simulink model "gm_FOC"  (R2020a)
settings: Solver=FixedStepAuto  StartTime=0.0  StopTime=10.0  RelTol=1e-3
libraries: hdlmdlgenlib x12
(part 1 of 2)
settings Model: Creator=black  LastModifiedBy=black
settings OptimizationCC: BlockReduction=off  ConditionallyExecuteInputs=off
settings DebuggingCC: InheritedTsInSrcMsg=none  SingleTaskRateTransMsg=error

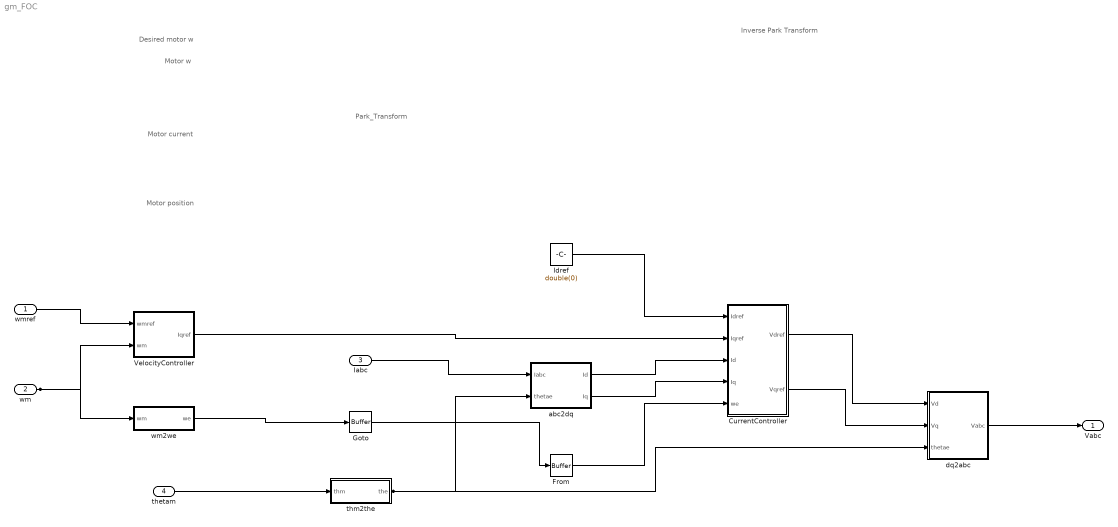
== system gm_FOC ==
  note: Motor position
  note: Motor current
  note: Desired motor w
  note: Motor w
  note: Park_Transform
  note: Inverse Park Transform
  wmref : Inport  OutDataTypeStr=double  Unit=rad/sec  PortDimensions=1  SampleTime=10000
  wm : Inport  Port=2  OutDataTypeStr=double  Unit=rad/sec  PortDimensions=1  SampleTime=10000
  Iabc : Inport  Port=3  OutDataTypeStr=single  Unit=A  PortDimensions=[3]  SampleTime=10000
  thetam : Inport  Port=4  OutDataTypeStr=double  Unit=rad  PortDimensions=1  SampleTime=10000
  CurrentController : Subsystem
  From : hdlmdlgenlib/Buffer
      settings: SourceProductBaseCode=SL
  Goto : hdlmdlgenlib/Buffer
      settings: SourceProductBaseCode=SL
  Idref : Constant  Value=double(0)  OutDataTypeStr=double  SampleTime=10000
  VelocityController : Subsystem
  abc2dq : Subsystem
  dq2abc : Subsystem
  thm2the : Subsystem
  wm2we : Subsystem
  Vabc : Outport  Unit=V  PortDimensions=3  VectorParamsAs1DForOutWhenUnconnected=off
  wires:
  wmref/1 -> VelocityController/1(wmref)
  wm/1 -> VelocityController/2(wm), wm2we/1(wm)
  Iabc/1 -> abc2dq/1(Iabc)
  thetam/1 -> thm2the/1(thm)
  CurrentController/1(Vdref) -> dq2abc/1(Vd)
  CurrentController/2(Vqref) -> dq2abc/2(Vq)
  From/1 -> CurrentController/5(we)
  Idref/1 -> CurrentController/1(Idref)
  VelocityController/1(Iqref) -> CurrentController/2(Iqref)
  abc2dq/1(Id) -> CurrentController/3(Id)
  abc2dq/2(Iq) -> CurrentController/4(Iq)
  dq2abc/1(Vabc) -> Vabc/1
  thm2the/1(the) -> abc2dq/2(thetae), dq2abc/3(thetae)
  wm2we/1(we) -> Goto/1
  Goto/1 -> From/1

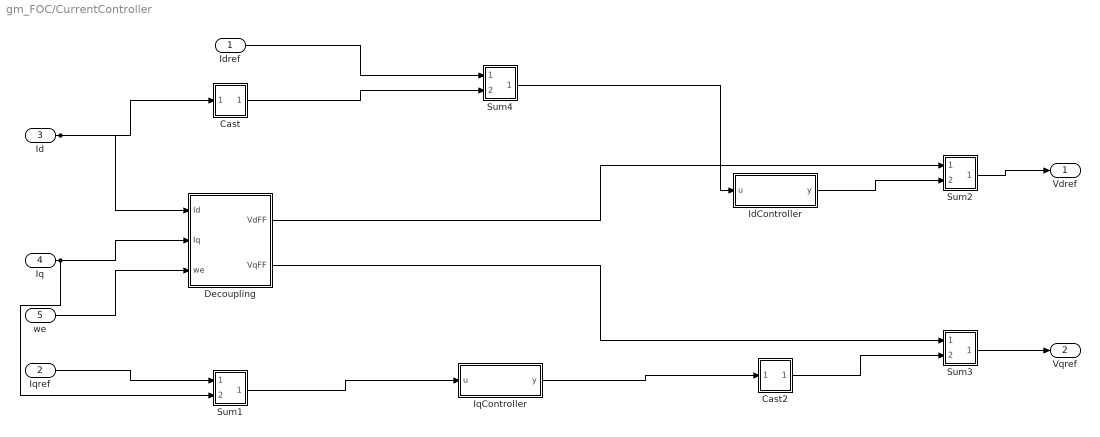
== system gm_FOC/CurrentController ==
  Idref : Inport  OutDataTypeStr=double  PortDimensions=1  SampleTime=10000
  Iqref : Inport  Port=2  OutDataTypeStr=single  PortDimensions=1  SampleTime=10000
  Id : Inport  Port=3  OutDataTypeStr=single  PortDimensions=1  SampleTime=10000
  Iq : Inport  Port=4  OutDataTypeStr=single  PortDimensions=1  SampleTime=10000
  we : Inport  Port=5  OutDataTypeStr=double  PortDimensions=1  SampleTime=10000
  Cast : Subsystem
      mask Display: disp('NFP\nconv');
  Cast2 : Subsystem
      mask Display: disp('NFP\nconv');
  Decoupling : Subsystem
  IdController : Subsystem
  IqController : Subsystem
  Sum1 : Subsystem
      mask Display: disp('NFP\nadd');
  Sum2 : Subsystem
      mask Display: disp('NFP\nadd');
  Sum3 : Subsystem
      mask Display: disp('NFP\nadd');
  Sum4 : Subsystem
      mask Display: disp('NFP\nadd');
  Vdref : Outport  VectorParamsAs1DForOutWhenUnconnected=off
  Vqref : Outport  Port=2  VectorParamsAs1DForOutWhenUnconnected=off
  wires:
  Idref/1 -> Sum4/1(In1)
  Iqref/1 -> Sum1/1(In1)
  Id/1 -> Cast/1(In1), Decoupling/1(Id)
  Iq/1 -> Sum1/2(In2), Decoupling/2(Iq)
  we/1 -> Decoupling/3(we)
  Decoupling/1(VdFF) -> Sum2/1(In1)
  Decoupling/2(VqFF) -> Sum3/1(In1)
  IdController/1(y) -> Sum2/2(In2)
  IqController/1(y) -> Cast2/1(In1)
  Cast/1(Out1) -> Sum4/2(In2)
  Cast2/1(Out1) -> Sum3/2(In2)
  Sum1/1(Out1) -> IqController/1(u)
  Sum2/1(Out1) -> Vdref/1
  Sum3/1(Out1) -> Vqref/1
  Sum4/1(Out1) -> IdController/1(u)

== system gm_FOC/VelocityController ==
  wmref : Inport  OutDataTypeStr=double  PortDimensions=1  SampleTime=10000
  wm : Inport  Port=2  OutDataTypeStr=double  PortDimensions=1  SampleTime=10000
  Cast : Subsystem
      mask Display: disp('NFP\nconv');
  Gain : Subsystem
      mask Display: disp('NFP\nmul');
  Gain_const : Constant  Value=single(3.3333332538604736)  OutDataTypeStr=single  SampleTime=10000
  PIDController : Subsystem
  Sum : Subsystem
      mask Display: disp('NFP\nadd');
  Iqref : Outport  VectorParamsAs1DForOutWhenUnconnected=off
  wires:
  wmref/1 -> Sum/1(In1)
  wm/1 -> Sum/2(In2)
  PIDController/1(y) -> Cast/1(In1)
  Gain_const/1 -> Gain/1(In1)
  Cast/1(Out1) -> Gain/2(In2)
  Sum/1(Out1) -> PIDController/1(u)
  Gain/1(Out1) -> Iqref/1

== system gm_FOC/abc2dq ==
  Iabc : Inport  OutDataTypeStr=single  PortDimensions=[3]  SampleTime=10000
  thetae : Inport  Port=2  OutDataTypeStr=single  PortDimensions=1  SampleTime=10000
  Park Transform : Subsystem  mask(Park Transform){AxisAlignment=D-axis, PowerInvariant=off}
      mask prompts: AxisAlignment "physmod:ee:library:comments:control:eeTransforms:PhaseaAxisAlignment_MP"; PowerInvariant "physmod:ee:library:comments:control:eeTransforms:PowerInvariant_MP"
      mask help: physmod:ee:library:comments:control:eeTransforms:ParkTransform_MD
      mask Help: web(nesl_help(gcbh))
      mask TypeOptions AxisAlignment: physmod:ee:library:comments:control:eeTransforms:Q0x2DAxis_PV | physmod:ee:library:comments:control:eeTransforms:D0x2DAxis_PV
      mask Display: ee.mask.drawParkTransform();
  Terminator : Terminator
  t : Demux  Outputs=3
  Id : Outport  VectorParamsAs1DForOutWhenUnconnected=off
  Iq : Outport  Port=2  VectorParamsAs1DForOutWhenUnconnected=off
  wires:
  Iabc/1 -> Park Transform/1(abc)
  thetae/1 -> Park Transform/2(theta)
  Park Transform/1(dq0) -> t/1
  t/1 -> Id/1
  t/2 -> Iq/1
  t/3 -> Terminator/1

== system gm_FOC/dq2abc ==
  Vd : Inport  OutDataTypeStr=double  PortDimensions=1  SampleTime=10000
  Vq : Inport  Port=2  OutDataTypeStr=double  PortDimensions=1  SampleTime=10000
  thetae : Inport  Port=3  OutDataTypeStr=single  PortDimensions=1  SampleTime=10000
  Cast : Subsystem
      mask Display: disp('NFP\nconv');
  Constant : Constant  Value=double(0)  OutDataTypeStr=double  SampleTime=10000
  Inverse Park Transform : Subsystem  mask(Inverse Park Transform){AxisAlignment=D-axis, PowerInvariant=off}
      mask prompts: AxisAlignment "physmod:ee:library:comments:control:eeTransforms:PhaseaAxisAlignment_MP"; PowerInvariant "physmod:ee:library:comments:control:eeTransforms:PowerInvariant_MP"
      mask help: physmod:ee:library:comments:control:eeTransforms:InverseParkTransform_MD
      mask Help: web(nesl_help(gcbh))
      mask TypeOptions AxisAlignment: physmod:ee:library:comments:control:eeTransforms:Q0x2DAxis_PV | physmod:ee:library:comments:control:eeTransforms:D0x2DAxis_PV
      mask Display: ee.mask.drawInverseParkTransform();
  mux : Mux  Inputs=3
  Vabc : Outport  Unit=V  PortDimensions=3  VectorParamsAs1DForOutWhenUnconnected=off
  wires:
  Vd/1 -> mux/1
  Vq/1 -> mux/2
  thetae/1 -> Inverse Park Transform/2(theta)
  Constant/1 -> mux/3
  Inverse Park Transform/1(abc) -> Vabc/1
  mux/1 -> Cast/1(In1)
  Cast/1(Out1) -> Inverse Park Transform/1(dq0)

== system gm_FOC/thm2the ==
  thm : Inport  OutDataTypeStr=double  PortDimensions=1  SampleTime=10000
  Cast : Subsystem
      mask Display: disp('NFP\nconv');
  Cast1 : Subsystem
      mask Display: disp('NFP\nconv');
  Constant : Constant  Value=double(6.283185307179586)  OutDataTypeStr=double  SampleTime=10000
  Mod : Subsystem
      mask Display: disp('NFP\nmath2');
  PolePairs : Subsystem
      mask Display: disp('NFP\ngain_pow2');
  the : Outport  VectorParamsAs1DForOutWhenUnconnected=off
  wires:
  thm/1 -> PolePairs/1(In1)
  Constant/1 -> Cast/1(In1)
  PolePairs/1(Out1) -> Cast1/1(In1)
  Cast/1(Out1) -> Mod/2(In2)
  Cast1/1(Out1) -> Mod/1(In1)
  Mod/1(Out1) -> the/1

== system gm_FOC/wm2we ==
  wm : Inport  OutDataTypeStr=double  PortDimensions=1  SampleTime=10000
  PolePairs : Subsystem
      mask Display: disp('NFP\ngain_pow2');
  we : Outport  VectorParamsAs1DForOutWhenUnconnected=off
  wires:
  wm/1 -> PolePairs/1(In1)
  PolePairs/1(Out1) -> we/1

== system gm_FOC/CurrentController/Cast ==
  In1 : Inport
  Cast : DataTypeConversion  OutDataTypeStr=double  RndMeth=Nearest  SampleTime=10000
  Out1 : Outport
  wires:
  In1/1 -> Cast/1
  Cast/1 -> Out1/1

== system gm_FOC/CurrentController/Cast2 ==
  In1 : Inport
  Cast2 : DataTypeConversion  OutDataTypeStr=double  RndMeth=Nearest  SampleTime=10000
  Out1 : Outport
  wires:
  In1/1 -> Cast2/1
  Cast2/1 -> Out1/1

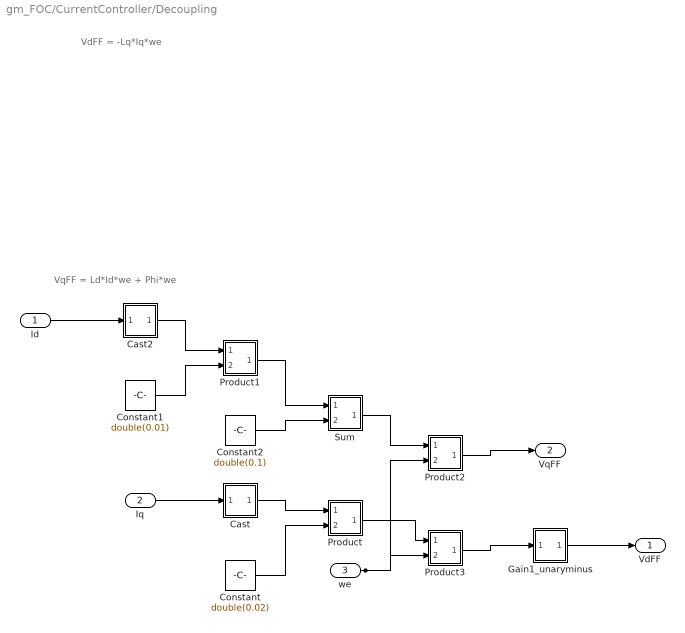
== system gm_FOC/CurrentController/Decoupling ==
  note: VdFF = -Lq*Iq*we
  note: VqFF = Ld*Id*we + Phi*we
  Id : Inport  OutDataTypeStr=single  PortDimensions=1  SampleTime=10000
  Iq : Inport  Port=2  OutDataTypeStr=single  PortDimensions=1  SampleTime=10000
  we : Inport  Port=3  OutDataTypeStr=double  PortDimensions=1  SampleTime=10000
  Cast : Subsystem
      mask Display: disp('NFP\nconv');
  Cast2 : Subsystem
      mask Display: disp('NFP\nconv');
  Constant : Constant  Value=double(0.02)  OutDataTypeStr=double  SampleTime=10000
  Constant1 : Constant  Value=double(0.01)  OutDataTypeStr=double  SampleTime=10000
  Constant2 : Constant  Value=double(0.1)  OutDataTypeStr=double  SampleTime=10000
  Gain1_unaryminus : Subsystem
      mask Display: disp('NFP\numinus');
  Product : Subsystem
      mask Display: disp('NFP\nmul');
  Product1 : Subsystem
      mask Display: disp('NFP\nmul');
  Product2 : Subsystem
      mask Display: disp('NFP\nmul');
  Product3 : Subsystem
      mask Display: disp('NFP\nmul');
  Sum : Subsystem
      mask Display: disp('NFP\nadd');
  VdFF : Outport  VectorParamsAs1DForOutWhenUnconnected=off
  VqFF : Outport  Port=2  VectorParamsAs1DForOutWhenUnconnected=off
  wires:
  Id/1 -> Cast2/1(In1)
  Iq/1 -> Cast/1(In1)
  we/1 -> Product3/2(In2), Product2/2(In2)
  Constant/1 -> Product/2(In2)
  Constant1/1 -> Product1/2(In2)
  Constant2/1 -> Sum/2(In2)
  Gain1_unaryminus/1(Out1) -> VdFF/1
  Cast/1(Out1) -> Product/1(In1)
  Cast2/1(Out1) -> Product1/1(In1)
  Product/1(Out1) -> Product3/1(In1)
  Product1/1(Out1) -> Sum/1(In1)
  Product2/1(Out1) -> VqFF/1
  Product3/1(Out1) -> Gain1_unaryminus/1(In1)
  Sum/1(Out1) -> Product2/1(In1)

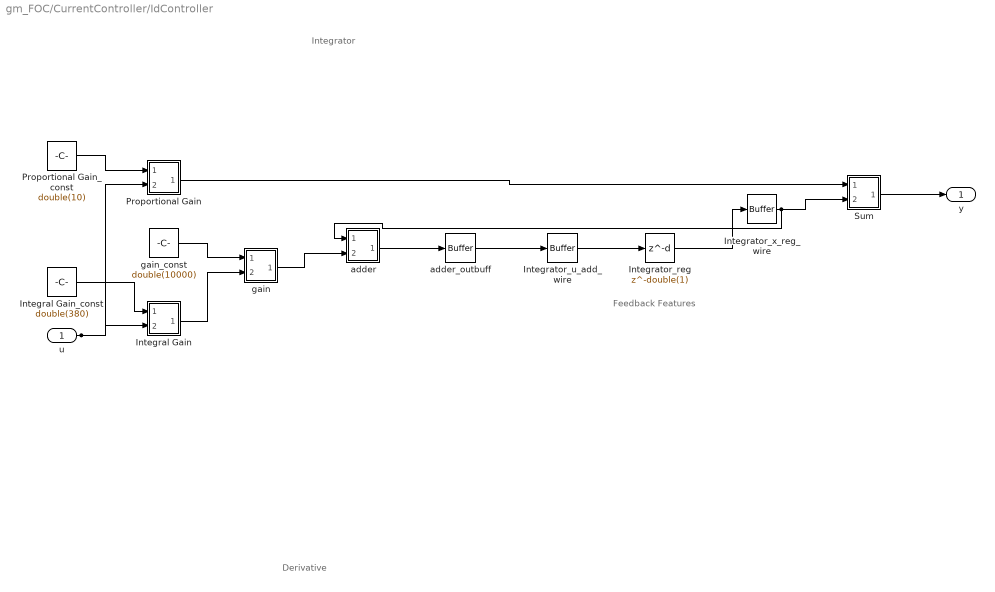
== system gm_FOC/CurrentController/IdController ==
  note: Feedback Features
  note: Derivative
  note: Integrator
  u : Inport  OutDataTypeStr=double  SampleTime=10000
  Integral Gain : Subsystem
      mask Display: disp('NFP\nmul');
  Integral Gain_const : Constant  Value=double(380)  OutDataTypeStr=double  SampleTime=10000
  Integrator_reg : Delay  DelayLength=double(1)  InitialCondition=0  SampleTime=10000
  Integrator_u_add_wire : hdlmdlgenlib/Buffer
      settings: SourceProductBaseCode=SL
  Integrator_x_reg_wire : hdlmdlgenlib/Buffer
      settings: SourceProductBaseCode=SL
  Proportional Gain : Subsystem
      mask Display: disp('NFP\nmul');
  Proportional Gain_const : Constant  Value=double(10)  OutDataTypeStr=double  SampleTime=10000
  Sum : Subsystem
      mask Display: disp('NFP\nadd');
  adder : Subsystem
      mask Display: disp('NFP\nadd');
  adder_outbuff : hdlmdlgenlib/Buffer
      settings: SourceProductBaseCode=SL
  gain : Subsystem
      mask Display: disp('NFP\nmul');
  gain_const : Constant  Value=double(10000)  OutDataTypeStr=double  SampleTime=10000
  y : Outport
  wires:
  u/1 -> Proportional Gain/2(In2), Integral Gain/2(In2)
  Integrator_x_reg_wire/1 -> Sum/2(In2), adder/1(In1)
  adder_outbuff/1 -> Integrator_u_add_wire/1
  Integrator_u_add_wire/1 -> Integrator_reg/1
  Integrator_reg/1 -> Integrator_x_reg_wire/1
  Integral Gain_const/1 -> Integral Gain/1(In1)
  gain_const/1 -> gain/1(In1)
  Proportional Gain_const/1 -> Proportional Gain/1(In1)
  adder/1(Out1) -> adder_outbuff/1
  Sum/1(Out1) -> y/1
  Integral Gain/1(Out1) -> gain/2(In2)
  gain/1(Out1) -> adder/2(In2)
  Proportional Gain/1(Out1) -> Sum/1(In1)

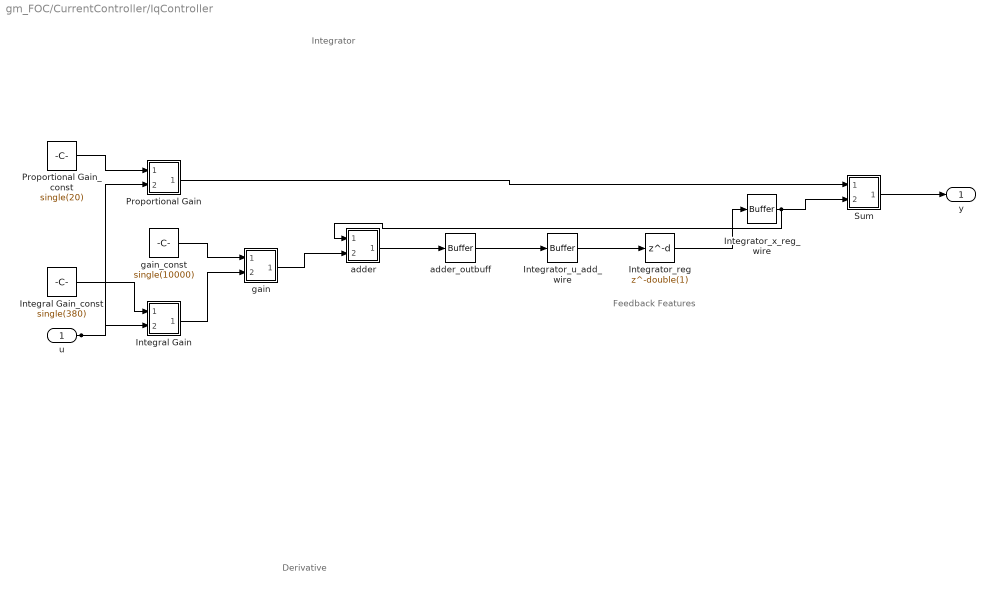
== system gm_FOC/CurrentController/IqController ==
  note: Feedback Features
  note: Derivative
  note: Integrator
  u : Inport  OutDataTypeStr=single  SampleTime=10000
  Integral Gain : Subsystem
      mask Display: disp('NFP\nmul');
  Integral Gain_const : Constant  Value=single(380)  OutDataTypeStr=single  SampleTime=10000
  Integrator_reg : Delay  DelayLength=double(1)  InitialCondition=0  SampleTime=10000
  Integrator_u_add_wire : hdlmdlgenlib/Buffer
      settings: SourceProductBaseCode=SL
  Integrator_x_reg_wire : hdlmdlgenlib/Buffer
      settings: SourceProductBaseCode=SL
  Proportional Gain : Subsystem
      mask Display: disp('NFP\nmul');
  Proportional Gain_const : Constant  Value=single(20)  OutDataTypeStr=single  SampleTime=10000
  Sum : Subsystem
      mask Display: disp('NFP\nadd');
  adder : Subsystem
      mask Display: disp('NFP\nadd');
  adder_outbuff : hdlmdlgenlib/Buffer
      settings: SourceProductBaseCode=SL
  gain : Subsystem
      mask Display: disp('NFP\nmul');
  gain_const : Constant  Value=single(10000)  OutDataTypeStr=single  SampleTime=10000
  y : Outport
  wires:
  u/1 -> Proportional Gain/2(In2), Integral Gain/2(In2)
  Integrator_x_reg_wire/1 -> Sum/2(In2), adder/1(In1)
  adder_outbuff/1 -> Integrator_u_add_wire/1
  Integrator_u_add_wire/1 -> Integrator_reg/1
  Integrator_reg/1 -> Integrator_x_reg_wire/1
  Integral Gain_const/1 -> Integral Gain/1(In1)
  gain_const/1 -> gain/1(In1)
  Proportional Gain_const/1 -> Proportional Gain/1(In1)
  adder/1(Out1) -> adder_outbuff/1
  Sum/1(Out1) -> y/1
  Integral Gain/1(Out1) -> gain/2(In2)
  gain/1(Out1) -> adder/2(In2)
  Proportional Gain/1(Out1) -> Sum/1(In1)

== system gm_FOC/CurrentController/Sum1 ==
  In1 : Inport
  In2 : Inport  Port=2
  Sum1 : Sum  Inputs=+-  OutDataTypeStr=single  SampleTime=10000
  Out1 : Outport
  wires:
  In1/1 -> Sum1/1
  In2/1 -> Sum1/2
  Sum1/1 -> Out1/1

== system gm_FOC/CurrentController/Sum2 ==
  In1 : Inport
  In2 : Inport  Port=2
  Sum2 : Sum  OutDataTypeStr=double  SampleTime=10000
  Out1 : Outport
  wires:
  In1/1 -> Sum2/1
  In2/1 -> Sum2/2
  Sum2/1 -> Out1/1

== system gm_FOC/CurrentController/Sum3 ==
  In1 : Inport
  In2 : Inport  Port=2
  Sum3 : Sum  OutDataTypeStr=double  SampleTime=10000
  Out1 : Outport
  wires:
  In1/1 -> Sum3/1
  In2/1 -> Sum3/2
  Sum3/1 -> Out1/1

== system gm_FOC/CurrentController/Sum4 ==
  In1 : Inport
  In2 : Inport  Port=2
  Sum4 : Sum  Inputs=+-  OutDataTypeStr=double  SampleTime=10000
  Out1 : Outport
  wires:
  In1/1 -> Sum4/1
  In2/1 -> Sum4/2
  Sum4/1 -> Out1/1

== system gm_FOC/VelocityController/Cast ==
  In1 : Inport
  Cast : DataTypeConversion  OutDataTypeStr=single  RndMeth=Nearest  SampleTime=10000
  Out1 : Outport
  wires:
  In1/1 -> Cast/1
  Cast/1 -> Out1/1

== system gm_FOC/VelocityController/Gain ==
  In1 : Inport
  In2 : Inport  Port=2
  Gain : Product  Inputs=**  OutDataTypeStr=single  SampleTime=10000
  Out1 : Outport
  wires:
  In1/1 -> Gain/1
  In2/1 -> Gain/2
  Gain/1 -> Out1/1

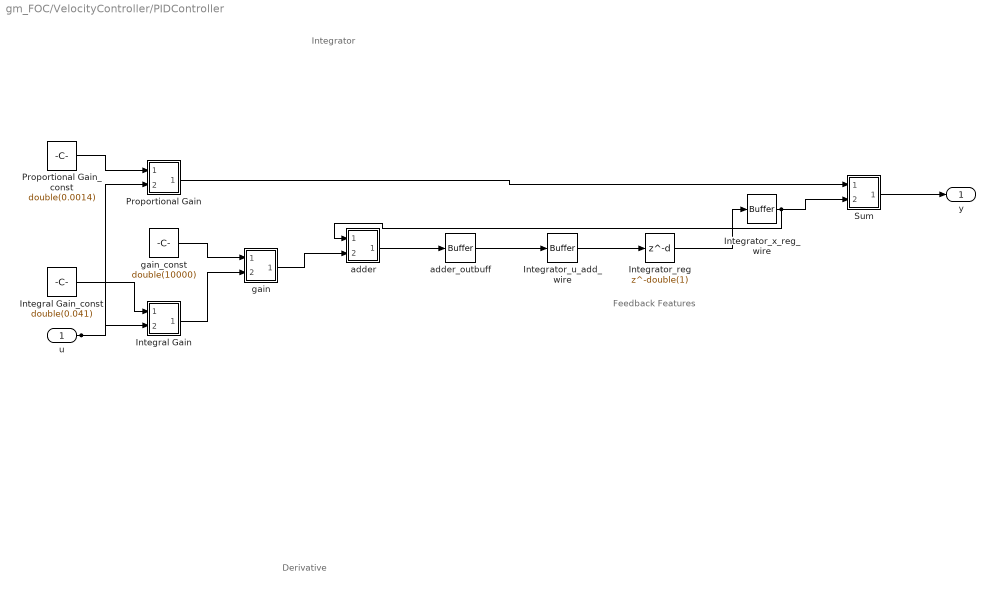
== system gm_FOC/VelocityController/PIDController ==
  note: Feedback Features
  note: Derivative
  note: Integrator
  u : Inport  OutDataTypeStr=double  SampleTime=10000
  Integral Gain : Subsystem
      mask Display: disp('NFP\nmul');
  Integral Gain_const : Constant  Value=double(0.041)  OutDataTypeStr=double  SampleTime=10000
  Integrator_reg : Delay  DelayLength=double(1)  InitialCondition=0  SampleTime=10000
  Integrator_u_add_wire : hdlmdlgenlib/Buffer
      settings: SourceProductBaseCode=SL
  Integrator_x_reg_wire : hdlmdlgenlib/Buffer
      settings: SourceProductBaseCode=SL
  Proportional Gain : Subsystem
      mask Display: disp('NFP\nmul');
  Proportional Gain_const : Constant  Value=double(0.0014)  OutDataTypeStr=double  SampleTime=10000
  Sum : Subsystem
      mask Display: disp('NFP\nadd');
  adder : Subsystem
      mask Display: disp('NFP\nadd');
  adder_outbuff : hdlmdlgenlib/Buffer
      settings: SourceProductBaseCode=SL
  gain : Subsystem
      mask Display: disp('NFP\nmul');
  gain_const : Constant  Value=double(10000)  OutDataTypeStr=double  SampleTime=10000
  y : Outport
  wires:
  u/1 -> Proportional Gain/2(In2), Integral Gain/2(In2)
  Integrator_x_reg_wire/1 -> Sum/2(In2), adder/1(In1)
  adder_outbuff/1 -> Integrator_u_add_wire/1
  Integrator_u_add_wire/1 -> Integrator_reg/1
  Integrator_reg/1 -> Integrator_x_reg_wire/1
  Integral Gain_const/1 -> Integral Gain/1(In1)
  gain_const/1 -> gain/1(In1)
  Proportional Gain_const/1 -> Proportional Gain/1(In1)
  adder/1(Out1) -> adder_outbuff/1
  Sum/1(Out1) -> y/1
  Integral Gain/1(Out1) -> gain/2(In2)
  gain/1(Out1) -> adder/2(In2)
  Proportional Gain/1(Out1) -> Sum/1(In1)

== system gm_FOC/VelocityController/Sum ==
  In1 : Inport
  In2 : Inport  Port=2
  Sum : Sum  Inputs=+-  OutDataTypeStr=double  SampleTime=10000
  Out1 : Outport
  wires:
  In1/1 -> Sum/1
  In2/1 -> Sum/2
  Sum/1 -> Out1/1

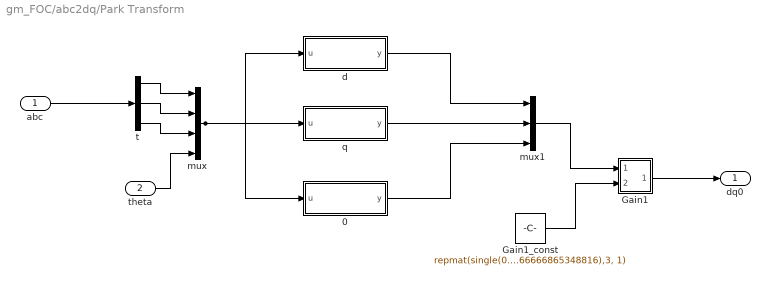
== system gm_FOC/abc2dq/Park Transform ==
  abc : Inport  OutDataTypeStr=single  PortDimensions=[3]  SampleTime=10000
  theta : Inport  Port=2  OutDataTypeStr=single  SampleTime=10000
  0 : Subsystem
  Gain1 : Subsystem
      mask Display: disp('NFP\nmul');
  Gain1_const : Constant  Value=repmat(single(0.6666666865348816),3, 1)  OutDataTypeStr=single  SampleTime=10000
  d : Subsystem
  mux : Mux
  mux1 : Mux  Inputs=3
  q : Subsystem
  t : Demux  Outputs=3
  dq0 : Outport
  wires:
  abc/1 -> t/1
  theta/1 -> mux/4
  0/1(y) -> mux1/3
  mux/1 -> q/1(u), d/1(u), 0/1(u)
  mux1/1 -> Gain1/1(In1)
  d/1(y) -> mux1/1
  q/1(y) -> mux1/2
  t/1 -> mux/1
  t/2 -> mux/2
  t/3 -> mux/3
  Gain1_const/1 -> Gain1/2(In2)
  Gain1/1(Out1) -> dq0/1

== system gm_FOC/dq2abc/Cast ==
  In1 : Inport
  Cast : DataTypeConversion  OutDataTypeStr=single  RndMeth=Nearest  SampleTime=10000
  Out1 : Outport
  wires:
  In1/1 -> Cast/1
  Cast/1 -> Out1/1

== system gm_FOC/dq2abc/Inverse Park Transform ==
  dq0 : Inport  OutDataTypeStr=single  PortDimensions=[3]  SampleTime=10000
  theta : Inport  Port=2  OutDataTypeStr=single  SampleTime=10000
  Gain1_unary : hdlmdlgenlib/Buffer
      settings: SourceProductBaseCode=SL
  a : Subsystem
  b : Subsystem
  c : Subsystem
  mux : Mux
  mux1 : Mux  Inputs=3
  t : Demux  Outputs=3
  abc : Outport
  wires:
  dq0/1 -> t/1
  theta/1 -> mux/4
  Gain1_unary/1 -> abc/1
  mux/1 -> c/1(u), b/1(u), a/1(u)
  mux1/1 -> Gain1_unary/1
  a/1(y) -> mux1/1
  b/1(y) -> mux1/2
  c/1(y) -> mux1/3
  t/1 -> mux/1
  t/2 -> mux/2
  t/3 -> mux/3

== system gm_FOC/thm2the/Cast ==
  In1 : Inport
  Cast : DataTypeConversion  OutDataTypeStr=single  RndMeth=Nearest  SampleTime=10000
  Out1 : Outport
  wires:
  In1/1 -> Cast/1
  Cast/1 -> Out1/1

== system gm_FOC/thm2the/Cast1 ==
  In1 : Inport
  Cast1 : DataTypeConversion  OutDataTypeStr=single  RndMeth=Nearest  SampleTime=10000
  Out1 : Outport
  wires:
  In1/1 -> Cast1/1
  Cast1/1 -> Out1/1

== system gm_FOC/thm2the/Mod ==
  In1 : Inport
  In2 : Inport  Port=2
  Mod : Math  Operator=mod  SampleTime=10000  SaturateOnIntegerOverflow=on
  Out1 : Outport
  wires:
  In1/1 -> Mod/1
  In2/1 -> Mod/2
  Mod/1 -> Out1/1

== system gm_FOC/thm2the/PolePairs ==
  In1 : Inport
  PolePairs : Gain  Gain=double(2)
  Out1 : Outport
  wires:
  In1/1 -> PolePairs/1
  PolePairs/1 -> Out1/1

== system gm_FOC/wm2we/PolePairs ==
  In1 : Inport
  PolePairs : Gain  Gain=double(2)
  Out1 : Outport
  wires:
  In1/1 -> PolePairs/1
  PolePairs/1 -> Out1/1

== system gm_FOC/CurrentController/Decoupling/Cast ==
  In1 : Inport
  Cast : DataTypeConversion  OutDataTypeStr=double  RndMeth=Nearest  SampleTime=10000
  Out1 : Outport
  wires:
  In1/1 -> Cast/1
  Cast/1 -> Out1/1

== system gm_FOC/CurrentController/Decoupling/Cast2 ==
  In1 : Inport
  Cast2 : DataTypeConversion  OutDataTypeStr=double  RndMeth=Nearest  SampleTime=10000
  Out1 : Outport
  wires:
  In1/1 -> Cast2/1
  Cast2/1 -> Out1/1

== system gm_FOC/CurrentController/Decoupling/Gain1_unaryminus ==
  In1 : Inport
  Gain1_unaryminus : UnaryMinus  SampleTime=10000
  Out1 : Outport
  wires:
  In1/1 -> Gain1_unaryminus/1
  Gain1_unaryminus/1 -> Out1/1

== system gm_FOC/CurrentController/Decoupling/Product ==
  In1 : Inport
  In2 : Inport  Port=2
  Product : Product  Inputs=**  OutDataTypeStr=double  SampleTime=10000
  Out1 : Outport
  wires:
  In1/1 -> Product/1
  In2/1 -> Product/2
  Product/1 -> Out1/1

== system gm_FOC/CurrentController/Decoupling/Product1 ==
  In1 : Inport
  In2 : Inport  Port=2
  Product1 : Product  Inputs=**  OutDataTypeStr=double  SampleTime=10000
  Out1 : Outport
  wires:
  In1/1 -> Product1/1
  In2/1 -> Product1/2
  Product1/1 -> Out1/1

== system gm_FOC/CurrentController/Decoupling/Product2 ==
  In1 : Inport
  In2 : Inport  Port=2
  Product2 : Product  Inputs=**  OutDataTypeStr=double  SampleTime=10000
  Out1 : Outport
  wires:
  In1/1 -> Product2/1
  In2/1 -> Product2/2
  Product2/1 -> Out1/1

== system gm_FOC/CurrentController/Decoupling/Product3 ==
  In1 : Inport
  In2 : Inport  Port=2
  Product3 : Product  Inputs=**  OutDataTypeStr=double  SampleTime=10000
  Out1 : Outport
  wires:
  In1/1 -> Product3/1
  In2/1 -> Product3/2
  Product3/1 -> Out1/1

== system gm_FOC/CurrentController/Decoupling/Sum ==
  In1 : Inport
  In2 : Inport  Port=2
  Sum : Sum  OutDataTypeStr=double  SampleTime=10000
  Out1 : Outport
  wires:
  In1/1 -> Sum/1
  In2/1 -> Sum/2
  Sum/1 -> Out1/1

== system gm_FOC/CurrentController/IdController/Integral Gain ==
  In1 : Inport
  In2 : Inport  Port=2
  Integral Gain : Product  Inputs=**  OutDataTypeStr=double  SampleTime=10000
  Out1 : Outport
  wires:
  In1/1 -> Integral Gain/1
  In2/1 -> Integral Gain/2
  Integral Gain/1 -> Out1/1

== system gm_FOC/CurrentController/IdController/Proportional Gain ==
  In1 : Inport
  In2 : Inport  Port=2
  Proportional Gain : Product  Inputs=**  OutDataTypeStr=double  SampleTime=10000
  Out1 : Outport
  wires:
  In1/1 -> Proportional Gain/1
  In2/1 -> Proportional Gain/2
  Proportional Gain/1 -> Out1/1

== system gm_FOC/CurrentController/IdController/Sum ==
  In1 : Inport
  In2 : Inport  Port=2
  Sum : Sum  OutDataTypeStr=double  SampleTime=10000
  Out1 : Outport
  wires:
  In1/1 -> Sum/1
  In2/1 -> Sum/2
  Sum/1 -> Out1/1

== system gm_FOC/CurrentController/IdController/adder ==
  In1 : Inport
  In2 : Inport  Port=2
  adder : Sum  OutDataTypeStr=double  SampleTime=10000
  Out1 : Outport
  wires:
  In1/1 -> adder/1
  In2/1 -> adder/2
  adder/1 -> Out1/1

== system gm_FOC/CurrentController/IdController/gain ==
  In1 : Inport
  In2 : Inport  Port=2
  gain : Product  Inputs=**  OutDataTypeStr=double  SampleTime=10000
  Out1 : Outport
  wires:
  In1/1 -> gain/1
  In2/1 -> gain/2
  gain/1 -> Out1/1

== system gm_FOC/CurrentController/IqController/Integral Gain ==
  In1 : Inport
  In2 : Inport  Port=2
  Integral Gain : Product  Inputs=**  OutDataTypeStr=single  SampleTime=10000
  Out1 : Outport
  wires:
  In1/1 -> Integral Gain/1
  In2/1 -> Integral Gain/2
  Integral Gain/1 -> Out1/1

== system gm_FOC/CurrentController/IqController/Proportional Gain ==
  In1 : Inport
  In2 : Inport  Port=2
  Proportional Gain : Product  Inputs=**  OutDataTypeStr=single  SampleTime=10000
  Out1 : Outport
  wires:
  In1/1 -> Proportional Gain/1
  In2/1 -> Proportional Gain/2
  Proportional Gain/1 -> Out1/1

== system gm_FOC/CurrentController/IqController/Sum ==
  In1 : Inport
  In2 : Inport  Port=2
  Sum : Sum  OutDataTypeStr=single  SampleTime=10000
  Out1 : Outport
  wires:
  In1/1 -> Sum/1
  In2/1 -> Sum/2
  Sum/1 -> Out1/1

== system gm_FOC/CurrentController/IqController/adder ==
  In1 : Inport
  In2 : Inport  Port=2
  adder : Sum  OutDataTypeStr=single  SampleTime=10000
  Out1 : Outport
  wires:
  In1/1 -> adder/1
  In2/1 -> adder/2
  adder/1 -> Out1/1

== system gm_FOC/CurrentController/IqController/gain ==
  In1 : Inport
  In2 : Inport  Port=2
  gain : Product  Inputs=**  OutDataTypeStr=single  SampleTime=10000
  Out1 : Outport
  wires:
  In1/1 -> gain/1
  In2/1 -> gain/2
  gain/1 -> Out1/1

== system gm_FOC/VelocityController/PIDController/Integral Gain ==
  In1 : Inport
  In2 : Inport  Port=2
  Integral Gain : Product  Inputs=**  OutDataTypeStr=double  SampleTime=10000
  Out1 : Outport
  wires:
  In1/1 -> Integral Gain/1
  In2/1 -> Integral Gain/2
  Integral Gain/1 -> Out1/1

== system gm_FOC/VelocityController/PIDController/Proportional Gain ==
  In1 : Inport
  In2 : Inport  Port=2
  Proportional Gain : Product  Inputs=**  OutDataTypeStr=double  SampleTime=10000
  Out1 : Outport
  wires:
  In1/1 -> Proportional Gain/1
  In2/1 -> Proportional Gain/2
  Proportional Gain/1 -> Out1/1

== system gm_FOC/VelocityController/PIDController/Sum ==
  In1 : Inport
  In2 : Inport  Port=2
  Sum : Sum  OutDataTypeStr=double  SampleTime=10000
  Out1 : Outport
  wires:
  In1/1 -> Sum/1
  In2/1 -> Sum/2
  Sum/1 -> Out1/1

== system gm_FOC/VelocityController/PIDController/adder ==
  In1 : Inport
  In2 : Inport  Port=2
  adder : Sum  OutDataTypeStr=double  SampleTime=10000
  Out1 : Outport
  wires:
  In1/1 -> adder/1
  In2/1 -> adder/2
  adder/1 -> Out1/1

== system gm_FOC/VelocityController/PIDController/gain ==
  In1 : Inport
  In2 : Inport  Port=2
  gain : Product  Inputs=**  OutDataTypeStr=double  SampleTime=10000
  Out1 : Outport
  wires:
  In1/1 -> gain/1
  In2/1 -> gain/2
  gain/1 -> Out1/1

== system gm_FOC/abc2dq/Park Transform/0 ==
  u : Inport  OutDataTypeStr=single  PortDimensions=[4 1]  SampleTime=10000
  Selector : Selector  SampleTime=10000  IndexOptions=Index vector (dialog)  Indices=double(1)  OutputSizes=double(0)
  Selector1 : Selector  SampleTime=10000  IndexOptions=Index vector (dialog)  Indices=double(2)  OutputSizes=double(0)
  Selector2 : Selector  SampleTime=10000  IndexOptions=Index vector (dialog)  Indices=double(3)  OutputSizes=double(0)
  adder : Subsystem
      mask Display: disp('NFP\nadd');
  adder1 : Subsystem
      mask Display: disp('NFP\nadd');
  gain : Subsystem
      mask Display: disp('NFP\ngain_pow2');
  y : Outport  OutDataTypeStr=single
  wires:
  u/1 -> Selector2/1, Selector1/1, Selector/1
  Selector/1 -> adder/1(In1)
  Selector1/1 -> adder/2(In2)
  Selector2/1 -> adder1/2(In2)
  adder/1(Out1) -> adder1/1(In1)
  adder1/1(Out1) -> gain/1(In1)
  gain/1(Out1) -> y/1

== system gm_FOC/abc2dq/Park Transform/Gain1 ==
  In1 : Inport
  In2 : Inport  Port=2
  Gain1 : Product  Inputs=**  OutDataTypeStr=single  SampleTime=10000
  Out1 : Outport
  wires:
  In1/1 -> Gain1/1
  In2/1 -> Gain1/2
  Gain1/1 -> Out1/1

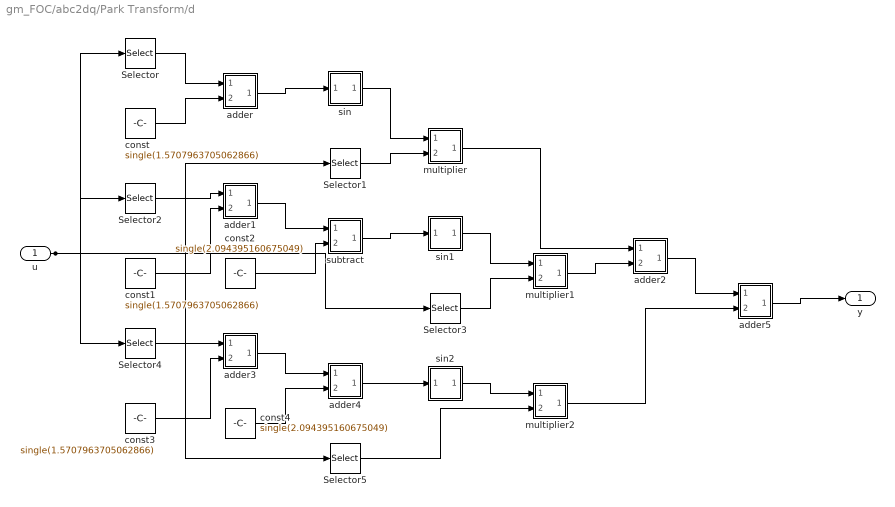
== system gm_FOC/abc2dq/Park Transform/d ==
  u : Inport  OutDataTypeStr=single  PortDimensions=[4 1]  SampleTime=10000
  Selector : Selector  SampleTime=10000  IndexOptions=Index vector (dialog)  Indices=double(4)  OutputSizes=double(0)
  Selector1 : Selector  SampleTime=10000  IndexOptions=Index vector (dialog)  Indices=double(1)  OutputSizes=double(0)
  Selector2 : Selector  SampleTime=10000  IndexOptions=Index vector (dialog)  Indices=double(4)  OutputSizes=double(0)
  Selector3 : Selector  SampleTime=10000  IndexOptions=Index vector (dialog)  Indices=double(2)  OutputSizes=double(0)
  Selector4 : Selector  SampleTime=10000  IndexOptions=Index vector (dialog)  Indices=double(4)  OutputSizes=double(0)
  Selector5 : Selector  SampleTime=10000  IndexOptions=Index vector (dialog)  Indices=double(3)  OutputSizes=double(0)
  adder : Subsystem
      mask Display: disp('NFP\nadd');
  adder1 : Subsystem
      mask Display: disp('NFP\nadd');
  adder2 : Subsystem
      mask Display: disp('NFP\nadd');
  adder3 : Subsystem
      mask Display: disp('NFP\nadd');
  adder4 : Subsystem
      mask Display: disp('NFP\nadd');
  adder5 : Subsystem
      mask Display: disp('NFP\nadd');
  const : Constant  Value=single(1.5707963705062866)  VectorParams1D=off  OutDataTypeStr=single  SampleTime=10000
  const1 : Constant  Value=single(1.5707963705062866)  VectorParams1D=off  OutDataTypeStr=single  SampleTime=10000
  const2 : Constant  Value=single(2.094395160675049)  VectorParams1D=off  OutDataTypeStr=single  SampleTime=10000
  const3 : Constant  Value=single(1.5707963705062866)  VectorParams1D=off  OutDataTypeStr=single  SampleTime=10000
  const4 : Constant  Value=single(2.094395160675049)  VectorParams1D=off  OutDataTypeStr=single  SampleTime=10000
  multiplier : Subsystem
      mask Display: disp('NFP\nmul');
  multiplier1 : Subsystem
      mask Display: disp('NFP\nmul');
  multiplier2 : Subsystem
      mask Display: disp('NFP\nmul');
  sin : Subsystem
      mask Display: disp('NFP\ntrig');
  sin1 : Subsystem
      mask Display: disp('NFP\ntrig');
  sin2 : Subsystem
      mask Display: disp('NFP\ntrig');
  subtract : Subsystem
      mask Display: disp('NFP\nadd');
  y : Outport  OutDataTypeStr=single
  wires:
  u/1 -> Selector5/1, Selector4/1, Selector3/1, Selector2/1, Selector1/1, Selector/1
  Selector/1 -> adder/1(In1)
  const/1 -> adder/2(In2)
  Selector1/1 -> multiplier/2(In2)
  Selector2/1 -> adder1/1(In1)
  const1/1 -> adder1/2(In2)
  const2/1 -> subtract/2(In2)
  Selector3/1 -> multiplier1/2(In2)
  Selector4/1 -> adder3/1(In1)
  const3/1 -> adder3/2(In2)
  const4/1 -> adder4/2(In2)
  Selector5/1 -> multiplier2/2(In2)
  adder/1(Out1) -> sin/1(In1)
  sin/1(Out1) -> multiplier/1(In1)
  multiplier/1(Out1) -> adder2/1(In1)
  adder1/1(Out1) -> subtract/1(In1)
  subtract/1(Out1) -> sin1/1(In1)
  sin1/1(Out1) -> multiplier1/1(In1)
  multiplier1/1(Out1) -> adder2/2(In2)
  adder2/1(Out1) -> adder5/1(In1)
  adder3/1(Out1) -> adder4/1(In1)
  adder4/1(Out1) -> sin2/1(In1)
  sin2/1(Out1) -> multiplier2/1(In1)
  multiplier2/1(Out1) -> adder5/2(In2)
  adder5/1(Out1) -> y/1

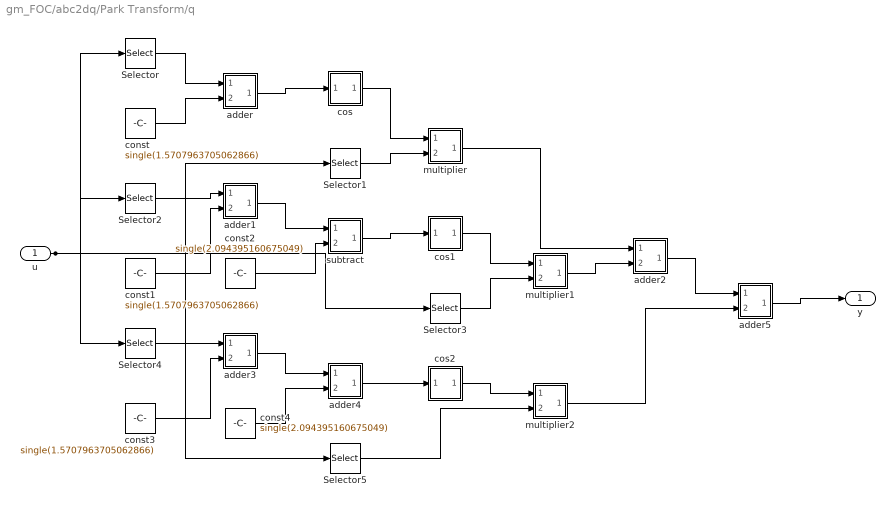
== system gm_FOC/abc2dq/Park Transform/q ==
  u : Inport  OutDataTypeStr=single  PortDimensions=[4 1]  SampleTime=10000
  Selector : Selector  SampleTime=10000  IndexOptions=Index vector (dialog)  Indices=double(4)  OutputSizes=double(0)
  Selector1 : Selector  SampleTime=10000  IndexOptions=Index vector (dialog)  Indices=double(1)  OutputSizes=double(0)
  Selector2 : Selector  SampleTime=10000  IndexOptions=Index vector (dialog)  Indices=double(4)  OutputSizes=double(0)
  Selector3 : Selector  SampleTime=10000  IndexOptions=Index vector (dialog)  Indices=double(2)  OutputSizes=double(0)
  Selector4 : Selector  SampleTime=10000  IndexOptions=Index vector (dialog)  Indices=double(4)  OutputSizes=double(0)
  Selector5 : Selector  SampleTime=10000  IndexOptions=Index vector (dialog)  Indices=double(3)  OutputSizes=double(0)
  adder : Subsystem
      mask Display: disp('NFP\nadd');
  adder1 : Subsystem
      mask Display: disp('NFP\nadd');
  adder2 : Subsystem
      mask Display: disp('NFP\nadd');
  adder3 : Subsystem
      mask Display: disp('NFP\nadd');
  adder4 : Subsystem
      mask Display: disp('NFP\nadd');
  adder5 : Subsystem
      mask Display: disp('NFP\nadd');
  const : Constant  Value=single(1.5707963705062866)  VectorParams1D=off  OutDataTypeStr=single  SampleTime=10000
  const1 : Constant  Value=single(1.5707963705062866)  VectorParams1D=off  OutDataTypeStr=single  SampleTime=10000
  const2 : Constant  Value=single(2.094395160675049)  VectorParams1D=off  OutDataTypeStr=single  SampleTime=10000
  const3 : Constant  Value=single(1.5707963705062866)  VectorParams1D=off  OutDataTypeStr=single  SampleTime=10000
  const4 : Constant  Value=single(2.094395160675049)  VectorParams1D=off  OutDataTypeStr=single  SampleTime=10000
  cos : Subsystem
      mask Display: disp('NFP\ntrig');
  cos1 : Subsystem
      mask Display: disp('NFP\ntrig');
  cos2 : Subsystem
      mask Display: disp('NFP\ntrig');
  multiplier : Subsystem
      mask Display: disp('NFP\nmul');
  multiplier1 : Subsystem
      mask Display: disp('NFP\nmul');
  multiplier2 : Subsystem
      mask Display: disp('NFP\nmul');
  subtract : Subsystem
      mask Display: disp('NFP\nadd');
  y : Outport  OutDataTypeStr=single
  wires:
  u/1 -> Selector5/1, Selector4/1, Selector3/1, Selector2/1, Selector1/1, Selector/1
  Selector/1 -> adder/1(In1)
  const/1 -> adder/2(In2)
  Selector1/1 -> multiplier/2(In2)
  Selector2/1 -> adder1/1(In1)
  const1/1 -> adder1/2(In2)
  const2/1 -> subtract/2(In2)
  Selector3/1 -> multiplier1/2(In2)
  Selector4/1 -> adder3/1(In1)
  const3/1 -> adder3/2(In2)
  const4/1 -> adder4/2(In2)
  Selector5/1 -> multiplier2/2(In2)
  adder/1(Out1) -> cos/1(In1)
  cos/1(Out1) -> multiplier/1(In1)
  multiplier/1(Out1) -> adder2/1(In1)
  adder1/1(Out1) -> subtract/1(In1)
  subtract/1(Out1) -> cos1/1(In1)
  cos1/1(Out1) -> multiplier1/1(In1)
  multiplier1/1(Out1) -> adder2/2(In2)
  adder2/1(Out1) -> adder5/1(In1)
  adder3/1(Out1) -> adder4/1(In1)
  adder4/1(Out1) -> cos2/1(In1)
  cos2/1(Out1) -> multiplier2/1(In1)
  multiplier2/1(Out1) -> adder5/2(In2)
  adder5/1(Out1) -> y/1

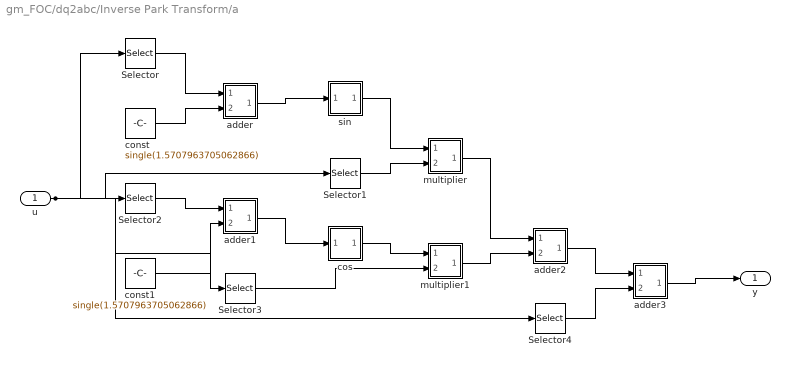
== system gm_FOC/dq2abc/Inverse Park Transform/a ==
  u : Inport  OutDataTypeStr=single  PortDimensions=[4 1]  SampleTime=10000
  Selector : Selector  SampleTime=10000  IndexOptions=Index vector (dialog)  Indices=double(4)  OutputSizes=double(0)
  Selector1 : Selector  SampleTime=10000  IndexOptions=Index vector (dialog)  Indices=double(1)  OutputSizes=double(0)
  Selector2 : Selector  SampleTime=10000  IndexOptions=Index vector (dialog)  Indices=double(4)  OutputSizes=double(0)
  Selector3 : Selector  SampleTime=10000  IndexOptions=Index vector (dialog)  Indices=double(2)  OutputSizes=double(0)
  Selector4 : Selector  SampleTime=10000  IndexOptions=Index vector (dialog)  Indices=double(3)  OutputSizes=double(0)
  adder : Subsystem
      mask Display: disp('NFP\nadd');
  adder1 : Subsystem
      mask Display: disp('NFP\nadd');
  adder2 : Subsystem
      mask Display: disp('NFP\nadd');
  adder3 : Subsystem
      mask Display: disp('NFP\nadd');
  const : Constant  Value=single(1.5707963705062866)  VectorParams1D=off  OutDataTypeStr=single  SampleTime=10000
  const1 : Constant  Value=single(1.5707963705062866)  VectorParams1D=off  OutDataTypeStr=single  SampleTime=10000
  cos : Subsystem
      mask Display: disp('NFP\ntrig');
  multiplier : Subsystem
      mask Display: disp('NFP\nmul');
  multiplier1 : Subsystem
      mask Display: disp('NFP\nmul');
  sin : Subsystem
      mask Display: disp('NFP\ntrig');
  y : Outport  OutDataTypeStr=single
  wires:
  u/1 -> Selector4/1, Selector3/1, Selector2/1, Selector1/1, Selector/1
  Selector/1 -> adder/1(In1)
  const/1 -> adder/2(In2)
  Selector1/1 -> multiplier/2(In2)
  Selector2/1 -> adder1/1(In1)
  const1/1 -> adder1/2(In2)
  Selector3/1 -> multiplier1/2(In2)
  Selector4/1 -> adder3/2(In2)
  adder/1(Out1) -> sin/1(In1)
  sin/1(Out1) -> multiplier/1(In1)
  multiplier/1(Out1) -> adder2/1(In1)
  adder1/1(Out1) -> cos/1(In1)
  cos/1(Out1) -> multiplier1/1(In1)
  multiplier1/1(Out1) -> adder2/2(In2)
  adder2/1(Out1) -> adder3/1(In1)
  adder3/1(Out1) -> y/1

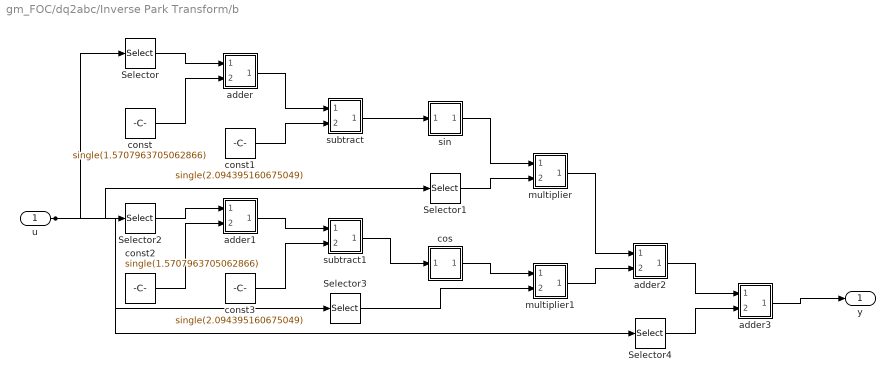
== system gm_FOC/dq2abc/Inverse Park Transform/b ==
  u : Inport  OutDataTypeStr=single  PortDimensions=[4 1]  SampleTime=10000
  Selector : Selector  SampleTime=10000  IndexOptions=Index vector (dialog)  Indices=double(4)  OutputSizes=double(0)
  Selector1 : Selector  SampleTime=10000  IndexOptions=Index vector (dialog)  Indices=double(1)  OutputSizes=double(0)
  Selector2 : Selector  SampleTime=10000  IndexOptions=Index vector (dialog)  Indices=double(4)  OutputSizes=double(0)
  Selector3 : Selector  SampleTime=10000  IndexOptions=Index vector (dialog)  Indices=double(2)  OutputSizes=double(0)
  Selector4 : Selector  SampleTime=10000  IndexOptions=Index vector (dialog)  Indices=double(3)  OutputSizes=double(0)
  adder : Subsystem
      mask Display: disp('NFP\nadd');
  adder1 : Subsystem
      mask Display: disp('NFP\nadd');
  adder2 : Subsystem
      mask Display: disp('NFP\nadd');
  adder3 : Subsystem
      mask Display: disp('NFP\nadd');
  const : Constant  Value=single(1.5707963705062866)  VectorParams1D=off  OutDataTypeStr=single  SampleTime=10000
  const1 : Constant  Value=single(2.094395160675049)  VectorParams1D=off  OutDataTypeStr=single  SampleTime=10000
  const2 : Constant  Value=single(1.5707963705062866)  VectorParams1D=off  OutDataTypeStr=single  SampleTime=10000
  const3 : Constant  Value=single(2.094395160675049)  VectorParams1D=off  OutDataTypeStr=single  SampleTime=10000
  cos : Subsystem
      mask Display: disp('NFP\ntrig');
  multiplier : Subsystem
      mask Display: disp('NFP\nmul');
  multiplier1 : Subsystem
      mask Display: disp('NFP\nmul');
  sin : Subsystem
      mask Display: disp('NFP\ntrig');
  subtract : Subsystem
      mask Display: disp('NFP\nadd');
  subtract1 : Subsystem
      mask Display: disp('NFP\nadd');
  y : Outport  OutDataTypeStr=single
  wires:
  u/1 -> Selector4/1, Selector3/1, Selector2/1, Selector1/1, Selector/1
  Selector/1 -> adder/1(In1)
  const/1 -> adder/2(In2)
  const1/1 -> subtract/2(In2)
  Selector1/1 -> multiplier/2(In2)
  Selector2/1 -> adder1/1(In1)
  const2/1 -> adder1/2(In2)
  const3/1 -> subtract1/2(In2)
  Selector3/1 -> multiplier1/2(In2)
  Selector4/1 -> adder3/2(In2)
  adder/1(Out1) -> subtract/1(In1)
  subtract/1(Out1) -> sin/1(In1)
  sin/1(Out1) -> multiplier/1(In1)
  multiplier/1(Out1) -> adder2/1(In1)
  adder1/1(Out1) -> subtract1/1(In1)
  subtract1/1(Out1) -> cos/1(In1)
  cos/1(Out1) -> multiplier1/1(In1)
  multiplier1/1(Out1) -> adder2/2(In2)
  adder2/1(Out1) -> adder3/1(In1)
  adder3/1(Out1) -> y/1

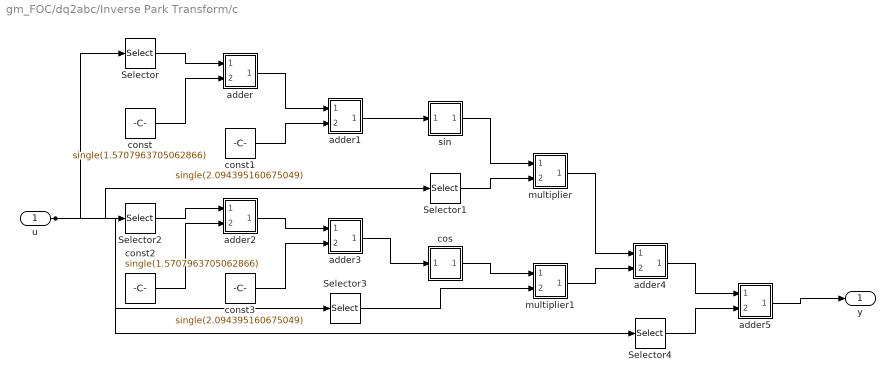
== system gm_FOC/dq2abc/Inverse Park Transform/c ==
  u : Inport  OutDataTypeStr=single  PortDimensions=[4 1]  SampleTime=10000
  Selector : Selector  SampleTime=10000  IndexOptions=Index vector (dialog)  Indices=double(4)  OutputSizes=double(0)
  Selector1 : Selector  SampleTime=10000  IndexOptions=Index vector (dialog)  Indices=double(1)  OutputSizes=double(0)
  Selector2 : Selector  SampleTime=10000  IndexOptions=Index vector (dialog)  Indices=double(4)  OutputSizes=double(0)
  Selector3 : Selector  SampleTime=10000  IndexOptions=Index vector (dialog)  Indices=double(2)  OutputSizes=double(0)
  Selector4 : Selector  SampleTime=10000  IndexOptions=Index vector (dialog)  Indices=double(3)  OutputSizes=double(0)
  adder : Subsystem
      mask Display: disp('NFP\nadd');
  adder1 : Subsystem
      mask Display: disp('NFP\nadd');
  adder2 : Subsystem
      mask Display: disp('NFP\nadd');
  adder3 : Subsystem
      mask Display: disp('NFP\nadd');
  adder4 : Subsystem
      mask Display: disp('NFP\nadd');
  adder5 : Subsystem
      mask Display: disp('NFP\nadd');
  const : Constant  Value=single(1.5707963705062866)  VectorParams1D=off  OutDataTypeStr=single  SampleTime=10000
  const1 : Constant  Value=single(2.094395160675049)  VectorParams1D=off  OutDataTypeStr=single  SampleTime=10000
  const2 : Constant  Value=single(1.5707963705062866)  VectorParams1D=off  OutDataTypeStr=single  SampleTime=10000
  const3 : Constant  Value=single(2.094395160675049)  VectorParams1D=off  OutDataTypeStr=single  SampleTime=10000
  cos : Subsystem
      mask Display: disp('NFP\ntrig');
  multiplier : Subsystem
      mask Display: disp('NFP\nmul');
  multiplier1 : Subsystem
      mask Display: disp('NFP\nmul');
  sin : Subsystem
      mask Display: disp('NFP\ntrig');
  y : Outport  OutDataTypeStr=single
  wires:
  u/1 -> Selector4/1, Selector3/1, Selector2/1, Selector1/1, Selector/1
  Selector/1 -> adder/1(In1)
  const/1 -> adder/2(In2)
  const1/1 -> adder1/2(In2)
  Selector1/1 -> multiplier/2(In2)
  Selector2/1 -> adder2/1(In1)
  const2/1 -> adder2/2(In2)
  const3/1 -> adder3/2(In2)
  Selector3/1 -> multiplier1/2(In2)
  Selector4/1 -> adder5/2(In2)
  adder/1(Out1) -> adder1/1(In1)
  adder1/1(Out1) -> sin/1(In1)
  sin/1(Out1) -> multiplier/1(In1)
  multiplier/1(Out1) -> adder4/1(In1)
  adder2/1(Out1) -> adder3/1(In1)
  adder3/1(Out1) -> cos/1(In1)
  cos/1(Out1) -> multiplier1/1(In1)
  multiplier1/1(Out1) -> adder4/2(In2)
  adder4/1(Out1) -> adder5/1(In1)
  adder5/1(Out1) -> y/1

== system gm_FOC/abc2dq/Park Transform/0/adder ==
  In1 : Inport
  In2 : Inport  Port=2
  adder : Sum  OutDataTypeStr=single  SampleTime=10000
  Out1 : Outport
  wires:
  In1/1 -> adder/1
  In2/1 -> adder/2
  adder/1 -> Out1/1

== system gm_FOC/abc2dq/Park Transform/0/adder1 ==
  In1 : Inport
  In2 : Inport  Port=2
  adder1 : Sum  OutDataTypeStr=single  SampleTime=10000
  Out1 : Outport
  wires:
  In1/1 -> adder1/1
  In2/1 -> adder1/2
  adder1/1 -> Out1/1

== system gm_FOC/abc2dq/Park Transform/0/gain ==
  In1 : Inport
  gain : Gain  Gain=single(0.5)
  Out1 : Outport
  wires:
  In1/1 -> gain/1
  gain/1 -> Out1/1

== system gm_FOC/abc2dq/Park Transform/d/adder ==
  In1 : Inport
  In2 : Inport  Port=2
  adder : Sum  OutDataTypeStr=single  SampleTime=10000
  Out1 : Outport
  wires:
  In1/1 -> adder/1
  In2/1 -> adder/2
  adder/1 -> Out1/1

== system gm_FOC/abc2dq/Park Transform/d/adder1 ==
  In1 : Inport
  In2 : Inport  Port=2
  adder1 : Sum  OutDataTypeStr=single  SampleTime=10000
  Out1 : Outport
  wires:
  In1/1 -> adder1/1
  In2/1 -> adder1/2
  adder1/1 -> Out1/1

== system gm_FOC/abc2dq/Park Transform/d/adder2 ==
  In1 : Inport
  In2 : Inport  Port=2
  adder2 : Sum  OutDataTypeStr=single  SampleTime=10000
  Out1 : Outport
  wires:
  In1/1 -> adder2/1
  In2/1 -> adder2/2
  adder2/1 -> Out1/1

== system gm_FOC/abc2dq/Park Transform/d/adder3 ==
  In1 : Inport
  In2 : Inport  Port=2
  adder3 : Sum  OutDataTypeStr=single  SampleTime=10000
  Out1 : Outport
  wires:
  In1/1 -> adder3/1
  In2/1 -> adder3/2
  adder3/1 -> Out1/1

== system gm_FOC/abc2dq/Park Transform/d/adder4 ==
  In1 : Inport
  In2 : Inport  Port=2
  adder4 : Sum  OutDataTypeStr=single  SampleTime=10000
  Out1 : Outport
  wires:
  In1/1 -> adder4/1
  In2/1 -> adder4/2
  adder4/1 -> Out1/1

== system gm_FOC/abc2dq/Park Transform/d/adder5 ==
  In1 : Inport
  In2 : Inport  Port=2
  adder5 : Sum  OutDataTypeStr=single  SampleTime=10000
  Out1 : Outport
  wires:
  In1/1 -> adder5/1
  In2/1 -> adder5/2
  adder5/1 -> Out1/1

== system gm_FOC/abc2dq/Park Transform/d/multiplier ==
  In1 : Inport
  In2 : Inport  Port=2
  multiplier : Product  Inputs=**  OutDataTypeStr=single  SampleTime=10000
  Out1 : Outport
  wires:
  In1/1 -> multiplier/1
  In2/1 -> multiplier/2
  multiplier/1 -> Out1/1

== system gm_FOC/abc2dq/Park Transform/d/multiplier1 ==
  In1 : Inport
  In2 : Inport  Port=2
  multiplier1 : Product  Inputs=**  OutDataTypeStr=single  SampleTime=10000
  Out1 : Outport
  wires:
  In1/1 -> multiplier1/1
  In2/1 -> multiplier1/2
  multiplier1/1 -> Out1/1

== system gm_FOC/abc2dq/Park Transform/d/multiplier2 ==
  In1 : Inport
  In2 : Inport  Port=2
  multiplier2 : Product  Inputs=**  OutDataTypeStr=single  SampleTime=10000
  Out1 : Outport
  wires:
  In1/1 -> multiplier2/1
  In2/1 -> multiplier2/2
  multiplier2/1 -> Out1/1

== system gm_FOC/abc2dq/Park Transform/d/sin ==
  In1 : Inport
  sin : Trigonometry  SampleTime=10000
  Out1 : Outport
  wires:
  In1/1 -> sin/1
  sin/1 -> Out1/1

== system gm_FOC/abc2dq/Park Transform/d/sin1 ==
  In1 : Inport
  sin1 : Trigonometry  SampleTime=10000
  Out1 : Outport
  wires:
  In1/1 -> sin1/1
  sin1/1 -> Out1/1

== system gm_FOC/abc2dq/Park Transform/d/sin2 ==
  In1 : Inport
  sin2 : Trigonometry  SampleTime=10000
  Out1 : Outport
  wires:
  In1/1 -> sin2/1
  sin2/1 -> Out1/1

== system gm_FOC/abc2dq/Park Transform/d/subtract ==
  In1 : Inport
  In2 : Inport  Port=2
  subtract : Sum  Inputs=+-  OutDataTypeStr=single  SampleTime=10000
  Out1 : Outport
  wires:
  In1/1 -> subtract/1
  In2/1 -> subtract/2
  subtract/1 -> Out1/1

== system gm_FOC/abc2dq/Park Transform/q/adder ==
  In1 : Inport
  In2 : Inport  Port=2
  adder : Sum  OutDataTypeStr=single  SampleTime=10000
  Out1 : Outport
  wires:
  In1/1 -> adder/1
  In2/1 -> adder/2
  adder/1 -> Out1/1

== system gm_FOC/abc2dq/Park Transform/q/adder1 ==
  In1 : Inport
  In2 : Inport  Port=2
  adder1 : Sum  OutDataTypeStr=single  SampleTime=10000
  Out1 : Outport
  wires:
  In1/1 -> adder1/1
  In2/1 -> adder1/2
  adder1/1 -> Out1/1

== system gm_FOC/abc2dq/Park Transform/q/adder2 ==
  In1 : Inport
  In2 : Inport  Port=2
  adder2 : Sum  OutDataTypeStr=single  SampleTime=10000
  Out1 : Outport
  wires:
  In1/1 -> adder2/1
  In2/1 -> adder2/2
  adder2/1 -> Out1/1

== system gm_FOC/abc2dq/Park Transform/q/adder3 ==
  In1 : Inport
  In2 : Inport  Port=2
  adder3 : Sum  OutDataTypeStr=single  SampleTime=10000
  Out1 : Outport
  wires:
  In1/1 -> adder3/1
  In2/1 -> adder3/2
  adder3/1 -> Out1/1

== system gm_FOC/abc2dq/Park Transform/q/adder4 ==
  In1 : Inport
  In2 : Inport  Port=2
  adder4 : Sum  OutDataTypeStr=single  SampleTime=10000
  Out1 : Outport
  wires:
  In1/1 -> adder4/1
  In2/1 -> adder4/2
  adder4/1 -> Out1/1

== system gm_FOC/abc2dq/Park Transform/q/adder5 ==
  In1 : Inport
  In2 : Inport  Port=2
  adder5 : Sum  OutDataTypeStr=single  SampleTime=10000
  Out1 : Outport
  wires:
  In1/1 -> adder5/1
  In2/1 -> adder5/2
  adder5/1 -> Out1/1

== system gm_FOC/abc2dq/Park Transform/q/cos ==
  In1 : Inport
  cos : Trigonometry  Operator=cos  SampleTime=10000
  Out1 : Outport
  wires:
  In1/1 -> cos/1
  cos/1 -> Out1/1

== system gm_FOC/abc2dq/Park Transform/q/cos1 ==
  In1 : Inport
  cos1 : Trigonometry  Operator=cos  SampleTime=10000
  Out1 : Outport
  wires:
  In1/1 -> cos1/1
  cos1/1 -> Out1/1

== system gm_FOC/abc2dq/Park Transform/q/cos2 ==
  In1 : Inport
  cos2 : Trigonometry  Operator=cos  SampleTime=10000
  Out1 : Outport
  wires:
  In1/1 -> cos2/1
  cos2/1 -> Out1/1

== system gm_FOC/abc2dq/Park Transform/q/multiplier ==
  In1 : Inport
  In2 : Inport  Port=2
  multiplier : Product  Inputs=**  OutDataTypeStr=single  SampleTime=10000
  Out1 : Outport
  wires:
  In1/1 -> multiplier/1
  In2/1 -> multiplier/2
  multiplier/1 -> Out1/1

== system gm_FOC/abc2dq/Park Transform/q/multiplier1 ==
  In1 : Inport
  In2 : Inport  Port=2
  multiplier1 : Product  Inputs=**  OutDataTypeStr=single  SampleTime=10000
  Out1 : Outport
  wires:
  In1/1 -> multiplier1/1
  In2/1 -> multiplier1/2
  multiplier1/1 -> Out1/1

== system gm_FOC/abc2dq/Park Transform/q/multiplier2 ==
  In1 : Inport
  In2 : Inport  Port=2
  multiplier2 : Product  Inputs=**  OutDataTypeStr=single  SampleTime=10000
  Out1 : Outport
  wires:
  In1/1 -> multiplier2/1
  In2/1 -> multiplier2/2
  multiplier2/1 -> Out1/1

== system gm_FOC/abc2dq/Park Transform/q/subtract ==
  In1 : Inport
  In2 : Inport  Port=2
  subtract : Sum  Inputs=+-  OutDataTypeStr=single  SampleTime=10000
  Out1 : Outport
  wires:
  In1/1 -> subtract/1
  In2/1 -> subtract/2
  subtract/1 -> Out1/1

== system gm_FOC/dq2abc/Inverse Park Transform/a/adder ==
  In1 : Inport
  In2 : Inport  Port=2
  adder : Sum  OutDataTypeStr=single  SampleTime=10000
  Out1 : Outport
  wires:
  In1/1 -> adder/1
  In2/1 -> adder/2
  adder/1 -> Out1/1

== system gm_FOC/dq2abc/Inverse Park Transform/a/adder1 ==
  In1 : Inport
  In2 : Inport  Port=2
  adder1 : Sum  OutDataTypeStr=single  SampleTime=10000
  Out1 : Outport
  wires:
  In1/1 -> adder1/1
  In2/1 -> adder1/2
  adder1/1 -> Out1/1

== system gm_FOC/dq2abc/Inverse Park Transform/a/adder2 ==
  In1 : Inport
  In2 : Inport  Port=2
  adder2 : Sum  OutDataTypeStr=single  SampleTime=10000
  Out1 : Outport
  wires:
  In1/1 -> adder2/1
  In2/1 -> adder2/2
  adder2/1 -> Out1/1

== system gm_FOC/dq2abc/Inverse Park Transform/a/adder3 ==
  In1 : Inport
  In2 : Inport  Port=2
  adder3 : Sum  OutDataTypeStr=single  SampleTime=10000
  Out1 : Outport
  wires:
  In1/1 -> adder3/1
  In2/1 -> adder3/2
  adder3/1 -> Out1/1

== system gm_FOC/dq2abc/Inverse Park Transform/a/cos ==
  In1 : Inport
  cos : Trigonometry  Operator=cos  SampleTime=10000
  Out1 : Outport
  wires:
  In1/1 -> cos/1
  cos/1 -> Out1/1

== system gm_FOC/dq2abc/Inverse Park Transform/a/multiplier ==
  In1 : Inport
  In2 : Inport  Port=2
  multiplier : Product  Inputs=**  OutDataTypeStr=single  SampleTime=10000
  Out1 : Outport
  wires:
  In1/1 -> multiplier/1
  In2/1 -> multiplier/2
  multiplier/1 -> Out1/1

== system gm_FOC/dq2abc/Inverse Park Transform/a/multiplier1 ==
  In1 : Inport
  In2 : Inport  Port=2
  multiplier1 : Product  Inputs=**  OutDataTypeStr=single  SampleTime=10000
  Out1 : Outport
  wires:
  In1/1 -> multiplier1/1
  In2/1 -> multiplier1/2
  multiplier1/1 -> Out1/1

== system gm_FOC/dq2abc/Inverse Park Transform/a/sin ==
  In1 : Inport
  sin : Trigonometry  SampleTime=10000
  Out1 : Outport
  wires:
  In1/1 -> sin/1
  sin/1 -> Out1/1

== system gm_FOC/dq2abc/Inverse Park Transform/b/adder ==
  In1 : Inport
  In2 : Inport  Port=2
  adder : Sum  OutDataTypeStr=single  SampleTime=10000
  Out1 : Outport
  wires:
  In1/1 -> adder/1
  In2/1 -> adder/2
  adder/1 -> Out1/1

== system gm_FOC/dq2abc/Inverse Park Transform/b/adder1 ==
  In1 : Inport
  In2 : Inport  Port=2
  adder1 : Sum  OutDataTypeStr=single  SampleTime=10000
  Out1 : Outport
  wires:
  In1/1 -> adder1/1
  In2/1 -> adder1/2
  adder1/1 -> Out1/1

== system gm_FOC/dq2abc/Inverse Park Transform/b/adder2 ==
  In1 : Inport
  In2 : Inport  Port=2
  adder2 : Sum  OutDataTypeStr=single  SampleTime=10000
  Out1 : Outport
  wires:
  In1/1 -> adder2/1
  In2/1 -> adder2/2
  adder2/1 -> Out1/1

== system gm_FOC/dq2abc/Inverse Park Transform/b/adder3 ==
  In1 : Inport
  In2 : Inport  Port=2
  adder3 : Sum  OutDataTypeStr=single  SampleTime=10000
  Out1 : Outport
  wires:
  In1/1 -> adder3/1
  In2/1 -> adder3/2
  adder3/1 -> Out1/1

== system gm_FOC/dq2abc/Inverse Park Transform/b/cos ==
  In1 : Inport
  cos : Trigonometry  Operator=cos  SampleTime=10000
  Out1 : Outport
  wires:
  In1/1 -> cos/1
  cos/1 -> Out1/1

== system gm_FOC/dq2abc/Inverse Park Transform/b/multiplier ==
  In1 : Inport
  In2 : Inport  Port=2
  multiplier : Product  Inputs=**  OutDataTypeStr=single  SampleTime=10000
  Out1 : Outport
  wires:
  In1/1 -> multiplier/1
  In2/1 -> multiplier/2
  multiplier/1 -> Out1/1

== system gm_FOC/dq2abc/Inverse Park Transform/b/multiplier1 ==
  In1 : Inport
  In2 : Inport  Port=2
  multiplier1 : Product  Inputs=**  OutDataTypeStr=single  SampleTime=10000
  Out1 : Outport
  wires:
  In1/1 -> multiplier1/1
  In2/1 -> multiplier1/2
  multiplier1/1 -> Out1/1

== system gm_FOC/dq2abc/Inverse Park Transform/b/sin ==
  In1 : Inport
  sin : Trigonometry  SampleTime=10000
  Out1 : Outport
  wires:
  In1/1 -> sin/1
  sin/1 -> Out1/1

== system gm_FOC/dq2abc/Inverse Park Transform/b/subtract ==
  In1 : Inport
  In2 : Inport  Port=2
  subtract : Sum  Inputs=+-  OutDataTypeStr=single  SampleTime=10000
  Out1 : Outport
  wires:
  In1/1 -> subtract/1
  In2/1 -> subtract/2
  subtract/1 -> Out1/1
